simulink model "SistemPrimerOrdeCont"  (R2015b)
settings: Solver=FixedStepAuto  SolverMode=SingleTasking  StartTime=-1*(1/1000)  StopTime=10*(1/1000)  FixedStep=100*(10^(-6))  RelTol=1e-3
settings Model: Creator=lukit  LastModifiedBy=lukit
settings DataIOCC: LimitDataPoints=off
settings DebuggingCC: AllowSymbolicDim=on  SFUnexpectedBacktrackingDiag=error  SFNoUnconditionalDefaultTransitionDiag=error
settings ModelReferenceCC: PropagateSignalLabelsOutOfModel=on
settings SFSimCC: SimUseLocalCustomCode=on
settings RTWCC: RTWUseLocalCustomCode=on
settings GRTTargetCC: TargetLangStandard=C99 (ISO)
settings ConfigComp: CovMetricSettings=dwe  CovHtmlReporting=off  CovSaveCumulativeToWorkspaceVar=off  CovSaveSingleToWorkspaceVar=off  CovModelRefEnable=Off  CovExternalEMLEnable=on

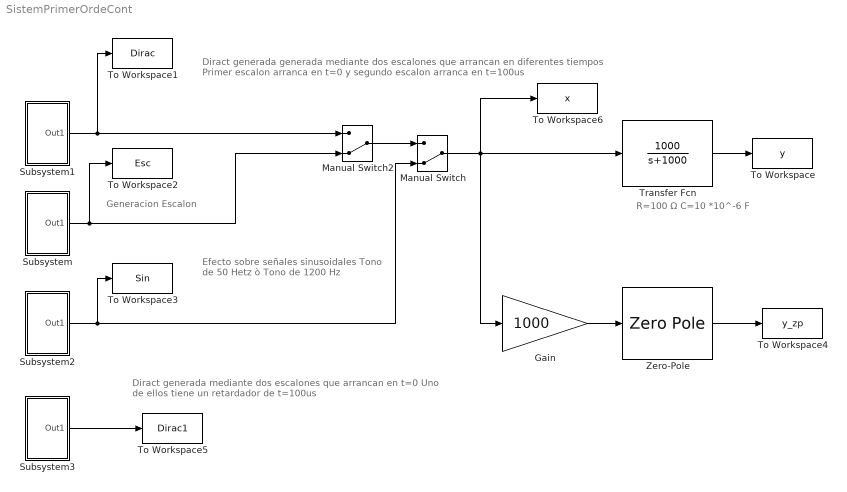
== system SistemPrimerOrdeCont ==
  note: R=100 Ω
      | C=10 *10^-6 F
  note: Generacion Escalon
  note: Diract generada generada mediante dos escalones que arrancan en diferentes tiempos
      | Primer escalon arranca en t=0 y segundo escalon arranca en t=100us
  note: Efecto sobre  señales sinusoidales
      | Tono de 50 Hetz ò Tono de 1200 Hz
  note: Diract generada mediante dos escalones que arrancan en t=0
      | Uno de ellos tiene un retardador de t=100us
  Gain : Gain  Gain=1000
  Manual Switch : ManualSwitch  CurrentSetting=0
  Manual Switch2 : ManualSwitch  CurrentSetting=0
  Subsystem : Subsystem
  Subsystem1 : Subsystem
  Subsystem2 : Subsystem
  Subsystem3 : Subsystem
  To Workspace : ToWorkspace  VariableName=y  SampleTime=-1
      settings: Save2DSignal=2-D array (concatenate along first dimension)
  To Workspace1 : ToWorkspace  VariableName=Dirac  SampleTime=-1
      settings: Save2DSignal=2-D array (concatenate along first dimension)
  To Workspace2 : ToWorkspace  VariableName=Esc  SampleTime=-1
      settings: Save2DSignal=2-D array (concatenate along first dimension)
  To Workspace3 : ToWorkspace  VariableName=Sin  SampleTime=-1
      settings: Save2DSignal=2-D array (concatenate along first dimension)
  To Workspace4 : ToWorkspace  VariableName=y_zp  SampleTime=-1
      settings: Save2DSignal=2-D array (concatenate along first dimension)
  To Workspace5 : ToWorkspace  VariableName=Dirac1  SampleTime=-1
      settings: Save2DSignal=2-D array (concatenate along first dimension)
  To Workspace6 : ToWorkspace  VariableName=x  SampleTime=-1
      settings: Save2DSignal=2-D array (concatenate along first dimension)
  Transfer Fcn : TransferFcn  Numerator=[0,1000]  Denominator=[1, 1000]
  Zero-Pole : ZeroPole  Zeros=[]  Poles=[-1000]
  wires:
  Manual Switch/1 -> Gain/1, Transfer Fcn/1, To Workspace6/1
  Transfer Fcn/1 -> To Workspace/1
  Subsystem/1(Out1) -> Manual Switch2/2, To Workspace2/1
  Subsystem1/1(Out1) -> To Workspace1/1, Manual Switch2/1
  Manual Switch2/1 -> Manual Switch/1
  Subsystem2/1(Out1) -> To Workspace3/1, Manual Switch/2
  Zero-Pole/1 -> To Workspace4/1
  Subsystem3/1(Out1) -> To Workspace5/1
  Gain/1 -> Zero-Pole/1

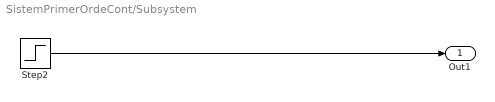
== system SistemPrimerOrdeCont/Subsystem ==
  Step2 : Step  Time=0
  Out1 : Outport
  wires:
  Step2/1 -> Out1/1

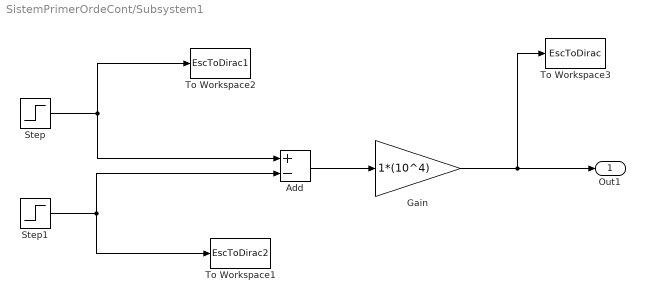
== system SistemPrimerOrdeCont/Subsystem1 ==
  Add : Sum  Inputs=+-
  Gain : Gain  Gain=1*(10^4)
  Step : Step  Time=0
  Step1 : Step  Time=100*10^(-6)
  To Workspace1 : ToWorkspace  VariableName=EscToDirac2  SampleTime=-1
      settings: Save2DSignal=2-D array (concatenate along first dimension)
  To Workspace2 : ToWorkspace  VariableName=EscToDirac1  SampleTime=-1
      settings: Save2DSignal=2-D array (concatenate along first dimension)
  To Workspace3 : ToWorkspace  VariableName=EscToDirac  SampleTime=-1
      settings: Save2DSignal=2-D array (concatenate along first dimension)
  Out1 : Outport
  wires:
  Step1/1 -> To Workspace1/1, Add/2
  Step/1 -> To Workspace2/1, Add/1
  Add/1 -> Gain/1
  Gain/1 -> To Workspace3/1, Out1/1

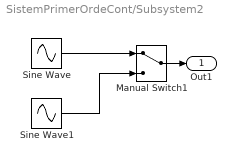
== system SistemPrimerOrdeCont/Subsystem2 ==
  Manual Switch1 : ManualSwitch
  Sine Wave : Sin  Frequency=2*pi*50
  Sine Wave1 : Sin  Frequency=2*pi*1200
  Out1 : Outport
  wires:
  Sine Wave/1 -> Manual Switch1/1
  Sine Wave1/1 -> Manual Switch1/2
  Manual Switch1/1 -> Out1/1

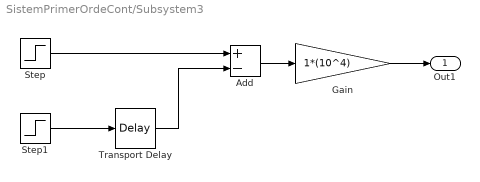
== system SistemPrimerOrdeCont/Subsystem3 ==
  Add : Sum  Inputs=+-
  Gain : Gain  Gain=1*(10^4)
  Step : Step  Time=0
  Step1 : Step  Time=0
  Transport Delay : TransportDelay  DelayTime=100*(10^(-6))  FixedBuffer=on
  Out1 : Outport
  wires:
  Step/1 -> Add/1
  Transport Delay/1 -> Add/2
  Step1/1 -> Transport Delay/1
  Add/1 -> Gain/1
  Gain/1 -> Out1/1
